simulink model "AccumulatorModel"  (R2020a)
settings: Solver=FixedStepAuto  StartTime=0.0  StopTime=330  FixedStep=1  RelTol=1e-2  AbsTol=1e-2
libraries: nesl_utility x14, LibGen_lib x5, fl_lib x4
settings Model: Creator=sean  LastModifiedBy=sean
settings SolverCC: AutoScaleAbsTol=off
settings DataIOCC: SignalLogging=off
settings OptimizationCC: DefaultParameterBehavior=Inlined  UseDivisionForNetSlopeComputation=on  GainParamInheritBuiltInType=on  UseFloatMulNetSlope=on  InlineInvariantSignals=on  PassReuseOutputArgsThreshold=0  EfficientFloat2IntCast=on  LifeSpan=1  OptimizeBlockOrder=speed  DifferentSizesBufferReuse=on
settings DebuggingCC: ParameterTunabilityLossMsg=error  SymbolicDimsDataTypeCodeGenerationDiagnostic=none  SFUnexpectedBacktrackingDiag=warning  SFNoUnconditionalDefaultTransitionDiag=warning
settings HardwareCC: ProdBitPerLong=64  ProdLongLongMode=on  ProdHWDeviceType=Intel->x86-64 (Linux 64)
settings SFSimCC: MATLABDynamicMemAlloc=off  CustomCodeUndefinedFunction=UseInterfaceOnly
settings RTWCC: Description=Generic Real-Time Target  GenCodeOnly=on  GenerateReport=on  BuildConfiguration=Faster Runs  LaunchReport=on
settings CodeAppCC: ForceParamTrailComments=on  OperatorAnnotations=on  EnableCustomComments=on
settings GRTTargetCC: CombineSignalStateStructs=on  MatFileLogging=off  SupportVariableSizeSignals=on
settings SimscapeCC: SimscapeLogDataHistory=10000

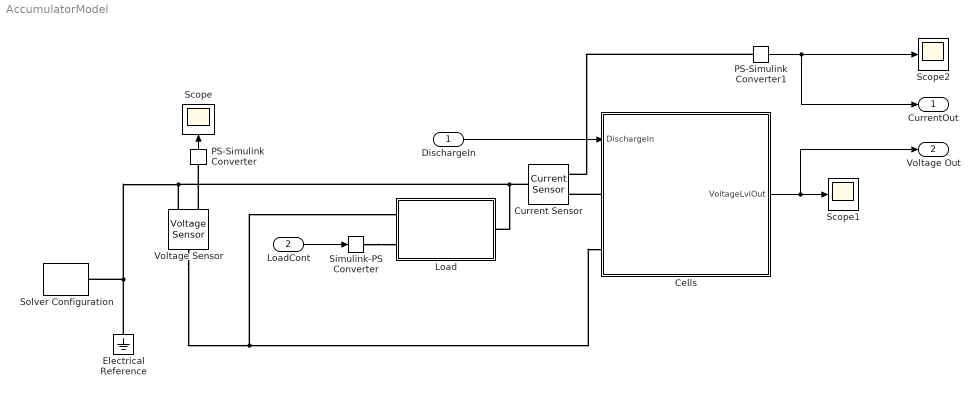
== system AccumulatorModel ==
  DischargeIn : Inport
  LoadCont : Inport  Port=2
  Cells : Subsystem
  Current Sensor : fl_lib/Electrical/Electrical Sensors/Current Sensor
  Electrical Reference : fl_lib/Electrical/Electrical Elements/Electrical Reference
  Load : Subsystem
  PS-Simulink Converter : nesl_utility/PS-Simulink Converter  PhysicalDomain=network_engine_domain  SubClassName=ps_output  LeftPortType=input  RightPortType=output  PseudoPeriodic=off  Frequencies=[]  Unit=inherit  AffineConversion=off
  PS-Simulink Converter1 : nesl_utility/PS-Simulink Converter  PhysicalDomain=network_engine_domain  SubClassName=ps_output  LeftPortType=input  RightPortType=output  PseudoPeriodic=off  Frequencies=[]  Unit=inherit  AffineConversion=off
  Scope : Scope
  Scope1 : Scope
  Scope2 : Scope
  Simulink-PS Converter : nesl_utility/Simulink-PS Converter  PhysicalDomain=network_engine_domain  SubClassName=ps_input  LeftPortType=input  RightPortType=output  PseudoPeriodic=off  Frequencies=[]  NoiseDistribution=none  NoiseParameters=[]  Unit=1  AffineConversion=off  FilteringAndDerivatives=provide  SimscapeFilterOrder=1  InputFilterTimeConstant=0.001  UdotUserProvided=0
  Solver Configuration : nesl_utility/Solver Configuration  PhysicalDomain=network_engine_domain  SubClassName=solver  LeftPortType=input  RightPortType=generic  Tones=[]  Harmonics=[]  SimulateNoise=off  Profile=off  UseLocalSampling=off  EnableSwitchedLinearOptims=on  FrequencyDomain=off  UseCCode=off  RelTol=0.001  AbsTol=1e-06  MinStep=1e-09  ToWorkspace=off  RevertToSquareIcSolve=off  NumHomotopyIterations=100  PhasorMode=off  PhasorModeNumHarmonics=1  DoDC=off  ResidualTolerance=1e-09  UseLocalSolver=off  LocalSolverChoice=NE_BACKWARD_EULER_ADVANCER  LocalSolverSampleTime=0.001  DoFixedCost=off  MaxNonlinIter=3  MaxModeIter=2  LinearAlgebra=auto  EquationFormulation=NE_TIME_EF  DelaysMemoryBudget=1024  AutomaticFiltering=on  FilteringTimeConstant=0.001  PartitionStorageMethod=AS_NEEDED  PartitionMemoryBudget=1024  PartitionMethod=ROBUST
  Voltage Sensor : fl_lib/Electrical/Electrical Sensors/Voltage Sensor
  CurrentOut : Outport
  Voltage Out : Outport  Port=2
  wires:
  PS-Simulink Converter/1 -> Scope/1
  Cells/1(VoltageLvlOut) -> Voltage Out/1, Scope1/1
  PS-Simulink Converter1/1 -> Scope2/1, CurrentOut/1
  DischargeIn/1 -> Cells/1(DischargeIn)
  LoadCont/1 -> Simulink-PS Converter/1
  connections:
  Electrical Reference/LConn1 -- Current Sensor/LConn1 -- Load/RConn1 -- Voltage Sensor/RConn2 -- Solver Configuration/RConn1
  Voltage Sensor/LConn1 -- Cells/LConn2 -- Load/LConn1
  Voltage Sensor/RConn1 -- PS-Simulink Converter/LConn1
  Cells/LConn1 -- Current Sensor/RConn2
  PS-Simulink Converter1/LConn1 -- Current Sensor/RConn1
  Simulink-PS Converter/RConn1 -- Load/LConn2

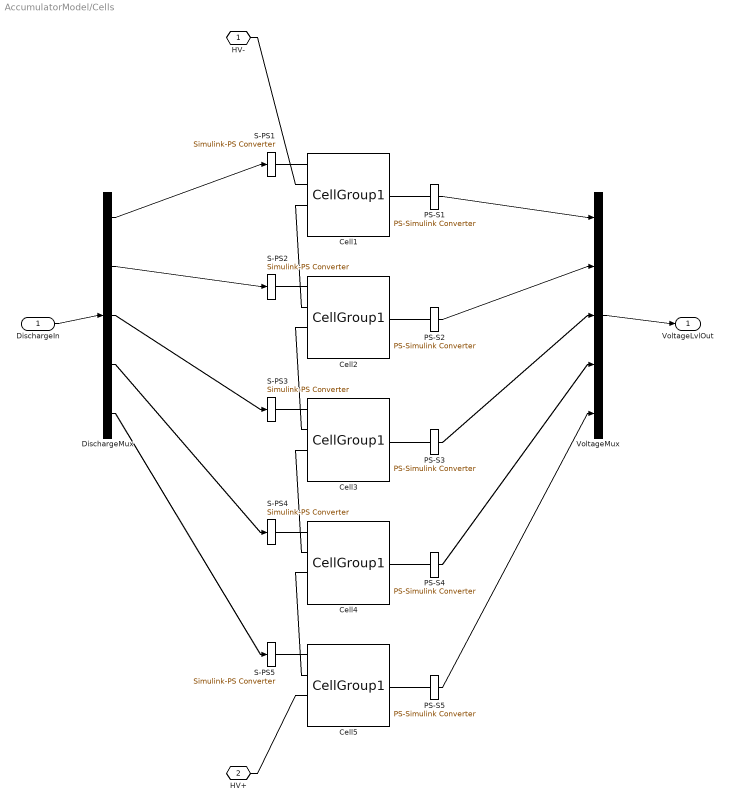
== system AccumulatorModel/Cells ==
  DischargeIn : Inport
  Cell1 : LibGen_lib/CellGroup1  Cell3StateOfCharge_specify=on  Cell3StateOfCharge_priority=High  Cell3StateOfCharge=0.7400  Cell3StateOfCharge_nominal_specify=off  Cell3StateOfCharge_nominal_unit=1  Cell3StateOfCharge_nominal_value=1  Cell2StateOfCharge_specify=on  Cell2StateOfCharge_priority=High  Cell2StateOfCharge=0.7400  Cell2StateOfCharge_nominal_specify=off  Cell2StateOfCharge_nominal_unit=1  Cell2StateOfCharge_nominal_value=1  Cell1StateOfCharge_specify=on  Cell1StateOfCharge_priority=High  Cell1StateOfCharge=0.7400  Cell1StateOfCharge_nominal_specify=off  Cell1StateOfCharge_nominal_unit=1  Cell1StateOfCharge_nominal_value=1
      settings: SourceProductName=Cell Library  InternalSimscapePortConfiguration="{\"Bottom\":[],\"Left\":[{\"id\":\"DischargeSig\",\"label\":\"DischargeSig\",\"type\":\"input\"},{\"id\":\"InConn\",\"label\":\"InConn\",\"type\":\"foundation.electrical.electrical\"},{\"id\":\"OutConn\",\"label\":\"OutConn\",\"type\":\"foundation.electrical.electrical\"},{\"id\":\"HeatConn\",\"label\":\"HeatConn\",\"type\":\"foundation.thermal.thermal\"}],\"Right\":[{\"id\":\"VoltageSig\",\"label\":\"VoltageSig\",\"type\":\"output\"}],\"Top\":[]}"
  Cell2 : LibGen_lib/CellGroup1  Cell3StateOfCharge_specify=on  Cell3StateOfCharge_priority=High  Cell3StateOfCharge=0.7400  Cell3StateOfCharge_nominal_specify=off  Cell3StateOfCharge_nominal_unit=1  Cell3StateOfCharge_nominal_value=1  Cell2StateOfCharge_specify=on  Cell2StateOfCharge_priority=High  Cell2StateOfCharge=0.7400  Cell2StateOfCharge_nominal_specify=off  Cell2StateOfCharge_nominal_unit=1  Cell2StateOfCharge_nominal_value=1  Cell1StateOfCharge_specify=on  Cell1StateOfCharge_priority=High  Cell1StateOfCharge=0.7400  Cell1StateOfCharge_nominal_specify=off  Cell1StateOfCharge_nominal_unit=1  Cell1StateOfCharge_nominal_value=1
      settings: SourceProductName=Cell Library  InternalSimscapePortConfiguration="{\"Bottom\":[],\"Left\":[{\"id\":\"DischargeSig\",\"label\":\"DischargeSig\",\"type\":\"input\"},{\"id\":\"InConn\",\"label\":\"InConn\",\"type\":\"foundation.electrical.electrical\"},{\"id\":\"OutConn\",\"label\":\"OutConn\",\"type\":\"foundation.electrical.electrical\"},{\"id\":\"HeatConn\",\"label\":\"HeatConn\",\"type\":\"foundation.thermal.thermal\"}],\"Right\":[{\"id\":\"VoltageSig\",\"label\":\"VoltageSig\",\"type\":\"output\"}],\"Top\":[]}"
  Cell3 : LibGen_lib/CellGroup1  Cell3StateOfCharge_specify=on  Cell3StateOfCharge_priority=High  Cell3StateOfCharge=0.7450  Cell3StateOfCharge_nominal_specify=off  Cell3StateOfCharge_nominal_unit=1  Cell3StateOfCharge_nominal_value=1  Cell2StateOfCharge_specify=on  Cell2StateOfCharge_priority=High  Cell2StateOfCharge=0.7450  Cell2StateOfCharge_nominal_specify=off  Cell2StateOfCharge_nominal_unit=1  Cell2StateOfCharge_nominal_value=1  Cell1StateOfCharge_specify=on  Cell1StateOfCharge_priority=High  Cell1StateOfCharge=0.7450  Cell1StateOfCharge_nominal_specify=off  Cell1StateOfCharge_nominal_unit=1  Cell1StateOfCharge_nominal_value=1
      settings: SourceProductName=Cell Library  InternalSimscapePortConfiguration="{\"Bottom\":[],\"Left\":[{\"id\":\"DischargeSig\",\"label\":\"DischargeSig\",\"type\":\"input\"},{\"id\":\"InConn\",\"label\":\"InConn\",\"type\":\"foundation.electrical.electrical\"},{\"id\":\"OutConn\",\"label\":\"OutConn\",\"type\":\"foundation.electrical.electrical\"},{\"id\":\"HeatConn\",\"label\":\"HeatConn\",\"type\":\"foundation.thermal.thermal\"}],\"Right\":[{\"id\":\"VoltageSig\",\"label\":\"VoltageSig\",\"type\":\"output\"}],\"Top\":[]}"
  Cell4 : LibGen_lib/CellGroup1  Cell3StateOfCharge_specify=on  Cell3StateOfCharge_priority=High  Cell3StateOfCharge=0.7480  Cell3StateOfCharge_nominal_specify=off  Cell3StateOfCharge_nominal_unit=1  Cell3StateOfCharge_nominal_value=1  Cell2StateOfCharge_specify=on  Cell2StateOfCharge_priority=High  Cell2StateOfCharge=0.7480  Cell2StateOfCharge_nominal_specify=off  Cell2StateOfCharge_nominal_unit=1  Cell2StateOfCharge_nominal_value=1  Cell1StateOfCharge_specify=on  Cell1StateOfCharge_priority=High  Cell1StateOfCharge=0.7480  Cell1StateOfCharge_nominal_specify=off  Cell1StateOfCharge_nominal_unit=1  Cell1StateOfCharge_nominal_value=1
      settings: SourceProductName=Cell Library  InternalSimscapePortConfiguration="{\"Bottom\":[],\"Left\":[{\"id\":\"DischargeSig\",\"label\":\"DischargeSig\",\"type\":\"input\"},{\"id\":\"InConn\",\"label\":\"InConn\",\"type\":\"foundation.electrical.electrical\"},{\"id\":\"OutConn\",\"label\":\"OutConn\",\"type\":\"foundation.electrical.electrical\"},{\"id\":\"HeatConn\",\"label\":\"HeatConn\",\"type\":\"foundation.thermal.thermal\"}],\"Right\":[{\"id\":\"VoltageSig\",\"label\":\"VoltageSig\",\"type\":\"output\"}],\"Top\":[]}"
  Cell5 : LibGen_lib/CellGroup1  Cell3StateOfCharge_specify=on  Cell3StateOfCharge_priority=High  Cell3StateOfCharge=0.7500  Cell3StateOfCharge_nominal_specify=off  Cell3StateOfCharge_nominal_unit=1  Cell3StateOfCharge_nominal_value=1  Cell2StateOfCharge_specify=on  Cell2StateOfCharge_priority=High  Cell2StateOfCharge=0.7500  Cell2StateOfCharge_nominal_specify=off  Cell2StateOfCharge_nominal_unit=1  Cell2StateOfCharge_nominal_value=1  Cell1StateOfCharge_specify=on  Cell1StateOfCharge_priority=High  Cell1StateOfCharge=0.7500  Cell1StateOfCharge_nominal_specify=off  Cell1StateOfCharge_nominal_unit=1  Cell1StateOfCharge_nominal_value=1
      settings: SourceProductName=Cell Library  InternalSimscapePortConfiguration="{\"Bottom\":[],\"Left\":[{\"id\":\"DischargeSig\",\"label\":\"DischargeSig\",\"type\":\"input\"},{\"id\":\"InConn\",\"label\":\"InConn\",\"type\":\"foundation.electrical.electrical\"},{\"id\":\"OutConn\",\"label\":\"OutConn\",\"type\":\"foundation.electrical.electrical\"},{\"id\":\"HeatConn\",\"label\":\"HeatConn\",\"type\":\"foundation.thermal.thermal\"}],\"Right\":[{\"id\":\"VoltageSig\",\"label\":\"VoltageSig\",\"type\":\"output\"}],\"Top\":[]}"
  DischargeMux : Demux  Outputs=5
  PS-S{1..5} (5 alike) : nesl_utility/PS-Simulink Converter  PhysicalDomain=network_engine_domain  SubClassName=ps_output  LeftPortType=input  RightPortType=output  PseudoPeriodic=off  Frequencies=[]  Unit=inherit  AffineConversion=off
  S-PS{1..5} (5 alike) : nesl_utility/Simulink-PS Converter  PhysicalDomain=network_engine_domain  SubClassName=ps_input  LeftPortType=input  RightPortType=output  PseudoPeriodic=off  Frequencies=[]  NoiseDistribution=none  NoiseParameters=[]  Unit=1  AffineConversion=off  FilteringAndDerivatives=provide  SimscapeFilterOrder=1  InputFilterTimeConstant=0.001  UdotUserProvided=0
  VoltageMux : Mux  Inputs=5
  HV- : PMIOPort  Side=Left
  HV+ : PMIOPort  Port=2  Side=Left
  VoltageLvlOut : Outport
  wires:
  DischargeMux/1 -> S-PS1/1
  PS-S1/1 -> VoltageMux/1
  DischargeMux/2 -> S-PS2/1
  PS-S2/1 -> VoltageMux/2
  DischargeMux/3 -> S-PS3/1
  PS-S3/1 -> VoltageMux/3
  DischargeMux/4 -> S-PS4/1
  PS-S4/1 -> VoltageMux/4
  DischargeMux/5 -> S-PS5/1
  PS-S5/1 -> VoltageMux/5
  DischargeIn/1 -> DischargeMux/1
  VoltageMux/1 -> VoltageLvlOut/1
  connections:
  S-PS1/RConn1 -- Cell1/LConn1
  PS-S1/LConn1 -- Cell1/RConn1
  S-PS2/RConn1 -- Cell2/LConn1
  PS-S2/LConn1 -- Cell2/RConn1
  Cell1/LConn3 -- Cell2/LConn2
  S-PS3/RConn1 -- Cell3/LConn1
  PS-S3/LConn1 -- Cell3/RConn1
  Cell2/LConn3 -- Cell3/LConn2
  S-PS4/RConn1 -- Cell4/LConn1
  PS-S4/LConn1 -- Cell4/RConn1
  Cell3/LConn3 -- Cell4/LConn2
  S-PS5/RConn1 -- Cell5/LConn1
  PS-S5/LConn1 -- Cell5/RConn1
  Cell4/LConn3 -- Cell5/LConn2
  Cell1/LConn2 -- HV-/RConn1
  Cell5/LConn3 -- HV+/RConn1

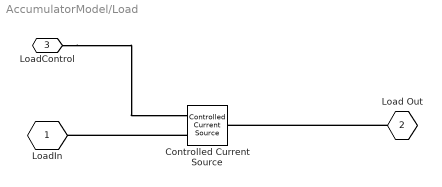
== system AccumulatorModel/Load ==
  Controlled Current Source : fl_lib/Electrical/Electrical Sources/Controlled Current Source
  LoadIn : PMIOPort  Tag=PMCPort  Side=Left
  Load Out : PMIOPort  Tag=PMCPort  Port=2  Side=Right
  LoadControl : PMIOPort  Port=3  Side=Left
  connections:
  Controlled Current Source/RConn2 -- LoadIn/RConn1
  Load Out/RConn1 -- Controlled Current Source/LConn1
  LoadControl/RConn1 -- Controlled Current Source/RConn1
